simulink model "NN_trajec_motion"  (R2016b)
settings: Solver=VariableStepAuto  StartTime=0.0  StopTime=20  RelTol=1e-3
undefined symbols (not defined in the file): X, Y, Z
libraries: neural x27, sm_lib x12, nesl_utility x9, simulink x6
(part 2 of 2)

== system NN_trajec_motion/Radial Basis Network1/Layer 1/Delays 1 ==
  "p{1}" : Inport  PortDimensions=6
      mask Display: e = 0.06;c1 = [120 230 180]/255;c2 = ([120 230 180]+0)/(256+128);c3 = ([120 230 180]+128)/(256+128);patch([0 1 1 0],[0 0 1 1],c1);patch([0 1 1 1-e 1-e 0+e],[0 0 1 1-e 0+e 0+e],c2);patch([0 0 1 1-e 0+e 0+e],[0 1 1 1-e 1-e 0+e],c3);plot([0 1 1 0 0],[0 0 1 1 0]);
  mux : Mux  Inputs=1
      mask Display: e = 0.06;c1 = [120 150 230]/255;c2 = ([120 150 230]+0)/383;c3 = ([120 150 230]+128)/383;patch([0 1 1 0],[0 0 1 1],c1);patch([0 1 1 1-e 1-e 0+e],[0 0 1 1-e 0+e 0+e],c2);patch([0 0 1 1-e 0+e 0+e],[0 1 1 1-e 1-e 0+e],c3);plot([0 1 1 0 0],[0 0 1 1 0]);disp('Mux')
  "pd{1,1}" : Outport
      mask Display: e = 0.06;c1 = [120 230 180]/255;c2 = ([120 230 180]+0)/(256+128);c3 = ([120 230 180]+128)/(256+128);patch([0 1 1 0],[0 0 1 1],c1);patch([0 1 1 1-e 1-e 0+e],[0 0 1 1-e 0+e 0+e],c2);patch([0 0 1 1-e 0+e 0+e],[0 1 1 1-e 1-e 0+e],c3);plot([0 1 1 0 0],[0 0 1 1 0]);
  wires:
  "p{1}"/1 -> mux/1
  mux/1 -> "pd{1,1}"/1

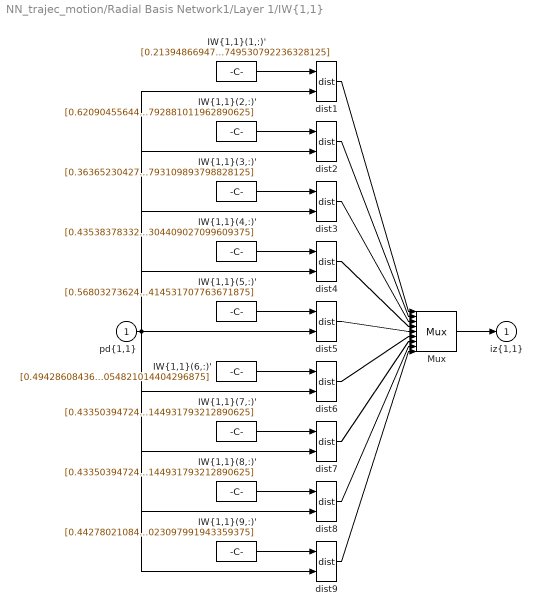
== system NN_trajec_motion/Radial Basis Network1/Layer 1/IW{1,1} ==
  "pd{1,1}" : Inport  PortDimensions=6
      mask Display: e = 0.06;c1 = [120 230 180]/255;c2 = ([120 230 180]+0)/(256+128);c3 = ([120 230 180]+128)/(256+128);patch([0 1 1 0],[0 0 1 1],c1);patch([0 1 1 1-e 1-e 0+e],[0 0 1 1-e 0+e 0+e],c2);patch([0 0 1 1-e 0+e 0+e],[0 1 1 1-e 1-e 0+e],c3);plot([0 1 1 0 0],[0 0 1 1 0]);
  "IW{1,1}(1,:)'" : Constant  Value=[0.21394866947440960291970668549765832722187042236328125;0.0801602817559704805550069295350112952291965484619140625;0.523334708212729537990526296198368072509765625;0.1711589355795276878868804715239093638956546783447265625;0.0641282254047763899951206667537917383015155792236328125;0.4186677665701836748013420219649560749530792236328125]
      mask Display: e = 0.06;c1 = [120 150 230]/255;c2 = ([120 150 230]+0)/383;c3 = ([120 150 230]+128)/383;patch([0 1 1 0],[0 0 1 1],c1);patch([0 1 1 1-e 1-e 0+e],[0 0 1 1-e 0+e 0+e],c2);patch([0 0 1 1-e 0+e 0+e],[0 1 1 1-e 1-e 0+e],c3);plot([0 1 1 0 0],[0 0 1 1 0]);disp('Weights');
  "IW{1,1}(2,:)'" : Constant  Value=[0.620904556442683830397299971082247793674468994140625;-0.136532993321228424132840473248506896197795867919921875;-0.478213928201944415974367075250484049320220947265625;0.4967236451541470199089189918595366179943084716796875;-0.10922639465698273653071481703591416589915752410888671875;-0.38257114256155555498395415270351804792881011962890625]
      mask Display: e = 0.06;c1 = [120 150 230]/255;c2 = ([120 150 230]+0)/383;c3 = ([120 150 230]+128)/383;patch([0 1 1 0],[0 0 1 1],c1);patch([0 1 1 1-e 1-e 0+e],[0 0 1 1-e 0+e 0+e],c2);patch([0 0 1 1-e 0+e 0+e],[0 1 1 1-e 1-e 0+e],c3);plot([0 1 1 0 0],[0 0 1 1 0]);disp('Weights');
  "IW{1,1}(3,:)'" : Constant  Value=[0.3636523042795689608652764945873059332370758056640625;0.10192237323971091444985148655177908949553966522216796875;0.258326477382186447950829233377589844167232513427734375;0.290921843423655179794451441921410150825977325439453125;0.08153789859176872878432362767853192053735256195068359375;0.2066611819057491417073180173247237689793109893798828125]
      mask Display: e = 0.06;c1 = [120 150 230]/255;c2 = ([120 150 230]+0)/383;c3 = ([120 150 230]+128)/383;patch([0 1 1 0],[0 0 1 1],c1);patch([0 1 1 1-e 1-e 0+e],[0 0 1 1-e 0+e 0+e],c2);patch([0 0 1 1-e 0+e 0+e],[0 1 1 1-e 1-e 0+e],c3);plot([0 1 1 0 0],[0 0 1 1 0]);disp('Weights');
  "IW{1,1}(4,:)'" : Constant  Value=[0.435383783322802198068046664047869853675365447998046875;0.059728018659380537058734006450322340242564678192138671875;-0.033420811038445845386757326878068852238357067108154296875;0.3483070266582417584544373312382958829402923583984375;0.0477824149275044296469872051602578721940517425537109375;-0.026736648830756680472742203846792108379304409027099609375]
      mask Display: e = 0.06;c1 = [120 150 230]/255;c2 = ([120 150 230]+0)/383;c3 = ([120 150 230]+128)/383;patch([0 1 1 0],[0 0 1 1],c1);patch([0 1 1 1-e 1-e 0+e],[0 0 1 1-e 0+e 0+e],c2);patch([0 0 1 1-e 0+e 0+e],[0 1 1 1-e 1-e 0+e],c3);plot([0 1 1 0 0],[0 0 1 1 0]);disp('Weights');
  "IW{1,1}(5,:)'" : Constant  Value=[0.5680327362483554853866962730535306036472320556640625;-0.055981432118557723776053336450786446221172809600830078125;-0.329950734387190858232230539215379394590854644775390625;0.45442618899868436610489652593969367444515228271484375;-0.0447851456948461790208426691606291569769382476806640625;-0.26396058750975270879024492387543432414531707763671875]
      mask Display: e = 0.06;c1 = [120 150 230]/255;c2 = ([120 150 230]+0)/383;c3 = ([120 150 230]+128)/383;patch([0 1 1 0],[0 0 1 1],c1);patch([0 1 1 1-e 1-e 0+e],[0 0 1 1-e 0+e 0+e],c2);patch([0 0 1 1-e 0+e 0+e],[0 1 1 1-e 1-e 0+e],c3);plot([0 1 1 0 0],[0 0 1 1 0]);disp('Weights');
  "IW{1,1}(6,:)'" : Constant  Value=[0.494286084363397104635140522077563218772411346435546875;-0.325483203772741813697422230688971467316150665283203125;-0.19346042345199399026256514844135381281375885009765625;0.39542886749071770591257291016518138349056243896484375;-0.260386563018193462060168030802742578089237213134765625;-0.1547683387615952088633974881304311566054821014404296875]
      mask Display: e = 0.06;c1 = [120 150 230]/255;c2 = ([120 150 230]+0)/383;c3 = ([120 150 230]+128)/383;patch([0 1 1 0],[0 0 1 1],c1);patch([0 1 1 1-e 1-e 0+e],[0 0 1 1-e 0+e 0+e],c2);patch([0 0 1 1-e 0+e 0+e],[0 1 1 1-e 1-e 0+e],c3);plot([0 1 1 0 0],[0 0 1 1 0]);disp('Weights');
  "IW{1,1}(7,:)'" : Constant  Value=[0.43350394724748053665308589188498444855213165283203125;0.29009857662759930274631869906443171203136444091796875;-0.140666868893681351604385554310283623635768890380859375;0.346803157797984429322468713507987558841705322265625;0.2320788613020794144414793436226318590342998504638671875;-0.112533495114945092385738689699792303144931793212890625]
      mask Display: e = 0.06;c1 = [120 150 230]/255;c2 = ([120 150 230]+0)/383;c3 = ([120 150 230]+128)/383;patch([0 1 1 0],[0 0 1 1],c1);patch([0 1 1 1-e 1-e 0+e],[0 0 1 1-e 0+e 0+e],c2);patch([0 0 1 1-e 0+e 0+e],[0 1 1 1-e 1-e 0+e],c3);plot([0 1 1 0 0],[0 0 1 1 0]);disp('Weights');
  "IW{1,1}(8,:)'" : Constant  Value=[0.43350394724748053665308589188498444855213165283203125;0.29009857662759930274631869906443171203136444091796875;-0.140666868893681351604385554310283623635768890380859375;0.346803157797984429322468713507987558841705322265625;0.2320788613020794144414793436226318590342998504638671875;-0.112533495114945092385738689699792303144931793212890625]
      mask Display: e = 0.06;c1 = [120 150 230]/255;c2 = ([120 150 230]+0)/383;c3 = ([120 150 230]+128)/383;patch([0 1 1 0],[0 0 1 1],c1);patch([0 1 1 1-e 1-e 0+e],[0 0 1 1-e 0+e 0+e],c2);patch([0 0 1 1-e 0+e 0+e],[0 1 1 1-e 1-e 0+e],c3);plot([0 1 1 0 0],[0 0 1 1 0]);disp('Weights');
  "IW{1,1}(9,:)'" : Constant  Value=[0.4427802108498635202948889855179004371166229248046875;0.053443047573277370487776494201170862652361392974853515625;-0.0620209863803692085237884157322696410119533538818359375;0.35422416867989081623591118841432034969329833984375;0.042754438058621897777999976142382365651428699493408203125;-0.049616789104295365431251951804370037280023097991943359375]
      mask Display: e = 0.06;c1 = [120 150 230]/255;c2 = ([120 150 230]+0)/383;c3 = ([120 150 230]+128)/383;patch([0 1 1 0],[0 0 1 1],c1);patch([0 1 1 1-e 1-e 0+e],[0 0 1 1-e 0+e 0+e],c2);patch([0 0 1 1-e 0+e 0+e],[0 1 1 1-e 1-e 0+e],c3);plot([0 1 1 0 0],[0 0 1 1 0]);disp('Weights');
  Mux : Mux  Inputs=9
      mask Display: e = 0.06;c1 = [120 150 230]/255;c2 = ([120 150 230]+0)/383;c3 = ([120 150 230]+128)/383;patch([0 1 1 0],[0 0 1 1],c1);patch([0 1 1 1-e 1-e 0+e],[0 0 1 1-e 0+e 0+e],c2);patch([0 0 1 1-e 0+e 0+e],[0 1 1 1-e 1-e 0+e],c3);plot([0 1 1 0 0],[0 0 1 1 0]);disp('Mux');
  dist{1..9} (9 alike) : neural/Weight Functions/dist
  "iz{1,1}" : Outport
      mask Display: e = 0.06;c1 = [120 230 180]/255;c2 = ([120 230 180]+0)/(256+128);c3 = ([120 230 180]+128)/(256+128);patch([0 1 1 0],[0 0 1 1],c1);patch([0 1 1 1-e 1-e 0+e],[0 0 1 1-e 0+e 0+e],c2);patch([0 0 1 1-e 0+e 0+e],[0 1 1 1-e 1-e 0+e],c3);plot([0 1 1 0 0],[0 0 1 1 0]);
  wires:
  "IW{1,1}(1,:)'"/1 -> dist1/1
  "pd{1,1}"/1 -> dist1/2, dist2/2, dist3/2, dist4/2, dist5/2, dist6/2, dist7/2, dist8/2, dist9/2
  dist1/1 -> Mux/1
  "IW{1,1}(2,:)'"/1 -> dist2/1
  dist2/1 -> Mux/2
  "IW{1,1}(3,:)'"/1 -> dist3/1
  dist3/1 -> Mux/3
  "IW{1,1}(4,:)'"/1 -> dist4/1
  dist4/1 -> Mux/4
  "IW{1,1}(5,:)'"/1 -> dist5/1
  dist5/1 -> Mux/5
  "IW{1,1}(6,:)'"/1 -> dist6/1
  dist6/1 -> Mux/6
  "IW{1,1}(7,:)'"/1 -> dist7/1
  dist7/1 -> Mux/7
  "IW{1,1}(8,:)'"/1 -> dist8/1
  dist8/1 -> Mux/8
  "IW{1,1}(9,:)'"/1 -> dist9/1
  dist9/1 -> Mux/9
  Mux/1 -> "iz{1,1}"/1

== system NN_trajec_motion/Radial Basis Network1/Layer 2/Delays 1 ==
  "p{2}" : Inport  PortDimensions=9
      mask Display: e = 0.06;c1 = [120 230 180]/255;c2 = ([120 230 180]+0)/(256+128);c3 = ([120 230 180]+128)/(256+128);patch([0 1 1 0],[0 0 1 1],c1);patch([0 1 1 1-e 1-e 0+e],[0 0 1 1-e 0+e 0+e],c2);patch([0 0 1 1-e 0+e 0+e],[0 1 1 1-e 1-e 0+e],c3);plot([0 1 1 0 0],[0 0 1 1 0]);
  mux : Mux  Inputs=1
      mask Display: e = 0.06;c1 = [120 150 230]/255;c2 = ([120 150 230]+0)/383;c3 = ([120 150 230]+128)/383;patch([0 1 1 0],[0 0 1 1],c1);patch([0 1 1 1-e 1-e 0+e],[0 0 1 1-e 0+e 0+e],c2);patch([0 0 1 1-e 0+e 0+e],[0 1 1 1-e 1-e 0+e],c3);plot([0 1 1 0 0],[0 0 1 1 0]);disp('Mux')
  "pd{2,1}" : Outport
      mask Display: e = 0.06;c1 = [120 230 180]/255;c2 = ([120 230 180]+0)/(256+128);c3 = ([120 230 180]+128)/(256+128);patch([0 1 1 0],[0 0 1 1],c1);patch([0 1 1 1-e 1-e 0+e],[0 0 1 1-e 0+e 0+e],c2);patch([0 0 1 1-e 0+e 0+e],[0 1 1 1-e 1-e 0+e],c3);plot([0 1 1 0 0],[0 0 1 1 0]);
  wires:
  "p{2}"/1 -> mux/1
  mux/1 -> "pd{2,1}"/1

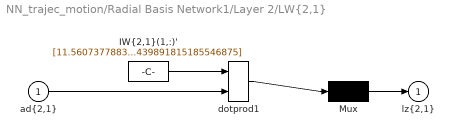
== system NN_trajec_motion/Radial Basis Network1/Layer 2/LW{2,1} ==
  "ad{2,1}" : Inport  PortDimensions=9
      mask Display: e = 0.06;c1 = [120 230 180]/255;c2 = ([120 230 180]+0)/(256+128);c3 = ([120 230 180]+128)/(256+128);patch([0 1 1 0],[0 0 1 1],c1);patch([0 1 1 1-e 1-e 0+e],[0 0 1 1-e 0+e 0+e],c2);patch([0 0 1 1-e 0+e 0+e],[0 1 1 1-e 1-e 0+e],c3);plot([0 1 1 0 0],[0 0 1 1 0]);
  "IW{2,1}(1,:)'" : Constant  Value=[11.560737788394089164967226679436862468719482421875;16.320936457119803009163661045022308826446533203125;4.10252576665253076981798585620708763599395751953125;-413.35195049574321046748082153499126434326171875;-58.50845415705041574483402655459940433502197265625;10.2011975993821568664543519844301044940948486328125;9.5186513478870580229340703226625919342041015625;0;427.41519974245665025591733865439891815185546875]
      mask Display: e = 0.06;c1 = [120 150 230]/255;c2 = ([120 150 230]+0)/383;c3 = ([120 150 230]+128)/383;patch([0 1 1 0],[0 0 1 1],c1);patch([0 1 1 1-e 1-e 0+e],[0 0 1 1-e 0+e 0+e],c2);patch([0 0 1 1-e 0+e 0+e],[0 1 1 1-e 1-e 0+e],c3);plot([0 1 1 0 0],[0 0 1 1 0]);disp('weights');
  Mux : Mux  Inputs=1
      mask Display: e = 0.06;c1 = [120 150 230]/255;c2 = ([120 150 230]+0)/383;c3 = ([120 150 230]+128)/383;patch([0 1 1 0],[0 0 1 1],c1);patch([0 1 1 1-e 1-e 0+e],[0 0 1 1-e 0+e 0+e],c2);patch([0 0 1 1-e 0+e 0+e],[0 1 1 1-e 1-e 0+e],c3);plot([0 1 1 0 0],[0 0 1 1 0]);disp('Mux');
  dotprod1 : neural/Weight Functions/dotprod
  "lz{2,1}" : Outport
      mask Display: e = 0.06;c1 = [120 230 180]/255;c2 = ([120 230 180]+0)/(256+128);c3 = ([120 230 180]+128)/(256+128);patch([0 1 1 0],[0 0 1 1],c1);patch([0 1 1 1-e 1-e 0+e],[0 0 1 1-e 0+e 0+e],c2);patch([0 0 1 1-e 0+e 0+e],[0 1 1 1-e 1-e 0+e],c3);plot([0 1 1 0 0],[0 0 1 1 0]);
  wires:
  "IW{2,1}(1,:)'"/1 -> dotprod1/1
  "ad{2,1}"/1 -> dotprod1/2
  dotprod1/1 -> Mux/1
  Mux/1 -> "lz{2,1}"/1

== matlab function NN_trajec_motion/G(q) ==
  data: q1 input; G output; q2 input
function G = fcn(q1,q2)
l1=0.41;% m
l2=0.39; % m
m1=2.34;%kg
m2=2.53;%kg
J1=0.76;%kgm^2
J2=0.69;%kgm^2
g=9.81;%kg/m^2
G=1/2*m1*g*l1*cos(q1*180/pi)+1/2*m2*g*l2*cos((q1+q2)*180/pi)+m2*g*l1*cos(q1*180/pi);
end

== matlab function NN_trajec_motion/M(q) ==
  data: M output; q1_dd input; q2 input; q2_dd input
function M = fcn(q1_dd,q2,q2_dd)
l1=0.41;% m
l2=0.39; % m
m1=2.34;%kg
m2=2.53;%kg
J1=0.76;%kgm^2
J2=0.69;%kgm^2
M=(J1+m2*l1^2+m2*l1*l2*cos(q2*180/pi)+J2)*q1_dd+(J2+1/2*m2*l1*l2*cos(q2*180/pi))*q2_dd;
end

== matlab function NN_trajec_motion/C(q,q') ==
  data: C output; q1_d input; q2 input; q2_d input
function C = fcn(q1_d,q2,q2_d)
l1=0.41;% m
l2=0.39; % m
m1=2.34;%kg
m2=2.53;%kg
J1=0.76;%kgm^2
J2=0.69;%kgm^2
C=(-1/2*m2*l1*l2*sin(q2*180/pi)*q2_d)*q1_d+(-1/2*m2*l1*l2*sin((q1_d+q2_d)*180/pi))*q2_d;
end

== matlab function NN_trajec_motion/C(q,q')1 ==
  data: q2 input; C1 output; q1_d input; q1_dd input
function C1 = fcn(q2,q1_d,q1_dd)
l1=0.41;% m
l2=0.39; % m
m1=2.34;%kg
m2=2.53;%kg
J1=0.76;%kgm^2
J2=0.69;%kgm^2
C1=1/2*m2*l1*l2*sin(q2*180/pi)*q1_d*q1_dd;
end

== matlab function NN_trajec_motion/G(q)1 ==
  data: q1 input; G1 output; q2 input
function G1 = fcn(q1,q2)
l1=0.41;% m
l2=0.39; % m
m1=2.34;%kg
m2=2.53;%kg
J1=0.76;%kgm^2
J2=0.69;%kgm^2
g=9.81;%kg/m^2
G1=1/2*m2*g*l2*cos((q1+q2)*180/pi);
end

== matlab function NN_trajec_motion/M(q)1 ==
  data: q1_dd input; M2 output; q2 input; q2_dd input
function M2 = fcn(q1_dd,q2,q2_dd)

l1=0.41;% m
l2=0.39; % m
m1=2.34;%kg
m2=2.53;%kg
J1=0.76;%kgm^2
J2=0.69;%kgm^2
M2=(J1+1/2*m2*l1*l2*cos(q2*180/pi))*q1_dd+J2*q2_dd;
end

== matlab function NN_trajec_motion/tao1_s=-ks*sgn(s) ==
  data: s input; tao1_s output
function tao1_s = fcn(s)
%% calculate the unknown disturbance
H=0.3;
t0_0=0;
T0_1=1.5;
T0_2=7;
t=0:0.01:20;
% S0
S_0=H/2*(1-cos(pi*(t-t0_0)/(T0_1-t0_0)));
t1_0=0;
T1_1=2;
T1_2=2;
H1=0.4;
% S21
S2_1=H1/2*(1-cos(pi*(t-t1_0)/(T1_1-t1_0)));
%S22 
S2_2=H1/2*(1-cos(pi*(t-T1_1-T1_2)/(T1_1-t1_0)));
% S3
t2_0=0;
T2_1=3;
T2_2=4;
H2=0.5;
% S31
S3_1=H2/2*(1-cos(pi*(t-t2_0)/(T2_1-t2_0)));
%S32 
S3_2=H2;
% S33 
S3_3=H2/2*(1-cos(pi*(t-T2_1-T2_2)/(T2_1-t2_0)));
a0=0.6;a21=0.6;a22=0.55;a31=0.35;a32=0.75;a33=0.35;
%% calculate ks
%ks=so+tao_d;so is the approximation error, tao_d is the unknown
%disturbance
tao_d=0.2*(a0*S_0+a21*S2_1+a22*S2_2+a31*S3_1+a32*S3_2+a33*S3_3);
s0=0.01;
Ks1=s0+tao_d;
tao1_s=-Ks1*sign(s);
end

== matlab function NN_trajec_motion/tao2_s=-ks2*sgn(s2) ==
  data: s2 input; tao2_s output
function tao2_s = fcn(s2)
%% calculate the unknown disturbance
H=0.3;
t0_0=0;
T0_1=1.5;
T0_2=7;
t=0:0.01:20;
% S0
S_0=H/2*(1-cos(pi*(t-t0_0)/(T0_1-t0_0)));
t1_0=0;
T1_1=2;
T1_2=2;
H1=0.4;
% S21
S2_1=H1/2*(1-cos(pi*(t-t1_0)/(T1_1-t1_0)));
%S22 
S2_2=H1/2*(1-cos(pi*(t-T1_1-T1_2)/(T1_1-t1_0)));
% S3
t2_0=0;
T2_1=3;
T2_2=4;
H2=0.5;
% S31
S3_1=H2/2*(1-cos(pi*(t-t2_0)/(T2_1-t2_0)));
%S32 
S3_2=H2;
% S33 
S3_3=H2/2*(1-cos(pi*(t-T2_1-T2_2)/(T2_1-t2_0)));
a0=0.6;a21=0.6;a22=0.55;a31=0.35;a32=0.75;a33=0.35;
%% calculate ks
%ks=so+tao_d;so is the approximation error, tao_d is the unknown
%disturbance
tao_d=0.2*(a0*S_0+a21*S2_1+a22*S2_2+a31*S3_1+a32*S3_2+a33*S3_3);
s0=0.01;
Ks2=s0+tao_d;
tao2_s=-Ks2*sign(s2);
end

== matlab function NN_trajec_motion/ RBF NN1 ==
  data: q1 input; q1_d input; q1_dd input; q2 input; q2_d input; q2_dd input; T11 output; qd1 input; qd2 input; qd1_d input; qd2_d input; qd1_dd input; qd2_dd input
function T11 = fcn(q1,q1_d,q1_dd,q2,q2_d,q2_dd,qd1,qd2,qd1_d,qd2_d,qd1_dd,qd2_dd)
l1=0.41;% m
l2=0.39; % m
m1=2.34;%kg
m2=2.53;%kg
J1=0.76;%kgm^2
J2=0.69;%kgm^2
g=9.81;%kg/m^2
tao1=(J1+m2*l1^2+m2*l1*l2*cos(q2)+J2)*q1_dd+(J2+1/2*m2*l1*l2*cos(q2))*q2_dd+...
    +(-1/2*m2*l1*l2*sin(q2)*q2_d)*q1_d+(-1/2*m2*l1*l2*sin((q1_d+q2_d)))*q2_d+...
    1/2*m1*g*l1*cos(q1)+1/2*m2*g*l2*cos((q1+q2))+m2*g*l1*cos(q1);
%using RBF network
P1=[q1;q1_d;q1_dd;q2;q2_d;q2_dd];
T1=tao1;
net_1=newrb(P1,T1,1e-2,1);

P11=[qd1;qd1_d;qd1_dd;qd2;qd2_d;qd2_dd];
T11=sim(net_1,P11);
end

== matlab function NN_trajec_motion/ RBF NN2 ==
  data: q1 input; q1_d input; q1_dd input; q2 input; q2_d input; q2_dd input; T22 output; qd1 input; qd2 input; qd1_d input; qd2_d input; qd1_dd input; qd2_dd input
function T22 = fcn(q1,q1_d,q1_dd,q2,q2_d,q2_dd,qd1,qd2,qd1_d,qd2_d,qd1_dd,qd2_dd)
l1=0.41;% m
l2=0.39; % m
m1=2.34;%kg
m2=2.53;%kg
J1=0.76;%kgm^2
J2=0.69;%kgm^2
g=9.81;%kg/m^2
tao2=(J1+1/2*m2*l1*l2*cos(q2*180/pi))*q1_dd+J2*q2_dd+...
    1/2*m2*l1*l2*sin(q2*180/pi)*q1_d*q1_dd+...
    1/2*m2*g*l2*cos((q1+q2)*180/pi);
%using RBF network
P2=[q1;q1_d;q1_dd;q2;q2_d;q2_dd];
T2=tao2;
net_2=newrb(P2,T2,1e-2,1);

P22=[qd1;qd1_d;qd1_dd;qd2;qd2_d;qd2_dd];
T22=sim(net_2,P22);
end
